simulink model "CELSIUS_A_FARENHEIT"  (R2024b)
settings: Solver=VariableStepAuto  StartTime=0.0  StopTime=20  RelTol=1e-3
libraries: simulink x1
settings Model: Creator=RREYM  LastModifiedBy=RREYM

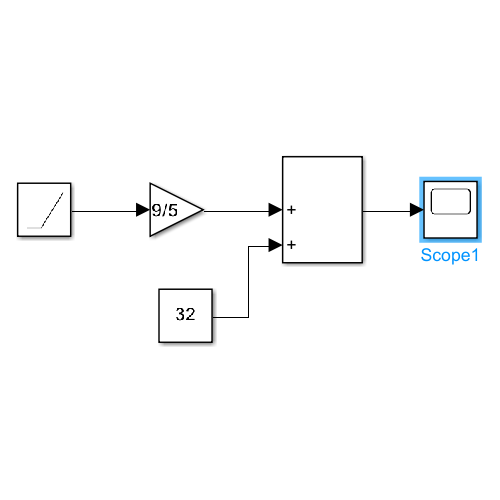
[thumbnail: Simulink's stored preview of the top-level diagram]
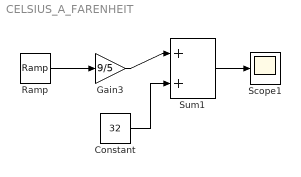
== system CELSIUS_A_FARENHEIT ==
  Constant : Constant  Value=32
  Gain3 : Gain  Gain=9/5
  Ramp : simulink/Sources/Ramp  slope=1  start=0  InitialOutput=0
  Scope1 : Scope
  Sum1 : Sum  Inputs=|++
  wires:
  Sum1/1 -> Scope1/1
  Constant/1 -> Sum1/2
  Gain3/1 -> Sum1/1
  Ramp/1 -> Gain3/1
